simulink model "A3_control_loop_tune"  (Simulink 8.7)
settings: Solver=ode45  StartTime=0.0  StopTime=5.0  MaxStep=1e-3  RelTol=1e-3
values from neighbouring files (symbols this model uses):
  b_1 = 2.39e6    (= 2390000)    [a1_main.m]    (also in a2_main.m; a3_main.m; a4_main.m)
  c_oil = 36.5e6    (= 36500000)    [a1_main.m]    (also in a2_main.m; a3_main.m; a4_main.m)
  c_p = 75e6    (= 75000000)    [a1_main.m]    (also in a2_main.m; a3_main.m; a4_main.m)
  K_M = 1/63000    (= 1.5873015873e-05)    [a1_main.m]    (also in a2_main.m; a3_main.m; a4_main.m)
  m_g = m_k + m_p    (= 268.7)    [a1_main.m]    (also in a2_main.m; a3_main.m; a4_main.m)
libraries: simulink x2
settings Model: Creator=jinyao  LastModifiedBy=jinyao
settings DataIOCC: LimitDataPoints=off  SaveFormat=Dataset
settings DebuggingCC: UnderspecifiedInitializationDetection=Simplified  MergeDetectMultiDrivingBlocksExec=error
settings HardwareCC: ProdBitPerPointer=64  ProdLargestAtomicFloat=Float  ProdIntDivRoundTo=Zero  ProdEndianess=LittleEndian  ProdWordSize=64  ProdHWDeviceType=Intel->x86-64 (Windows64)
settings ModelReferenceCC: PropagateSignalLabelsOutOfModel=on
settings ConfigComp: CovModelRefEnable=off

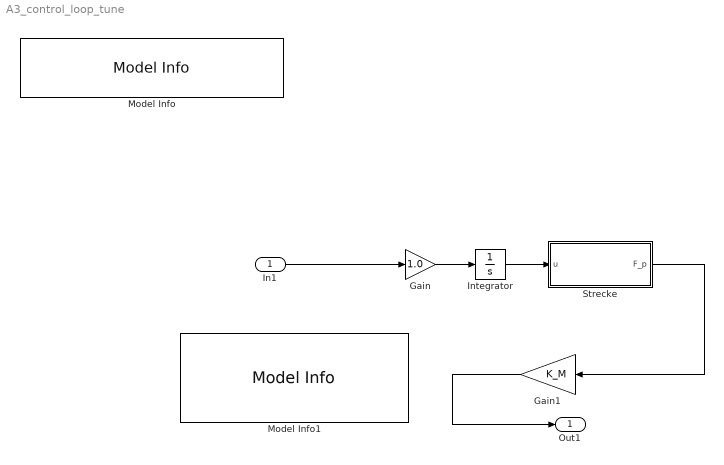
== system A3_control_loop_tune ==
  In1 : Inport
  Gain : Gain  Gain=1.0
  Gain1 : Gain  Gain=K_M
  Integrator : Integrator
  Model Info : simulink/Model-Wide Utilities/Model Info  Frame=on  DisplayStringWithTags=|  HorizontalTextAlignment=Center  LeftAlignmentValue=0.5  SourceBlockDiagram=A3_control_loop_tune  TagMaxNumber=20
      | %<ModelName>
      | 
      | GRUPPE 11
      | 
      | Cao,Bozhi  Gao,Yue  Jia,Xuehua  Zhu,Jinyao
  Model Info1 : simulink/Model-Wide Utilities/Model Info  Frame=on  DisplayStringWithTags=|  HorizontalTextAlignment=Center  LeftAlignmentValue=0.5  SourceBlockDiagram=A3_control_loop_tune  TagMaxNumber=20
      | %<ModelName>
      | 
      | MODSIM GRUPPE 11
      | 
      | Cao,Bozhi  Gao,Yue  Jia,Xuehua  Zhu,Jinyao
      | 
      | 14.06.2018
  Strecke : Subsystem
  Out1 : Outport
  wires:
  Integrator/1 -> Strecke/1(u)
  Gain/1 -> Integrator/1
  In1/1 -> Gain/1
  Strecke/1(F_p) -> Gain1/1
  Gain1/1 -> Out1/1

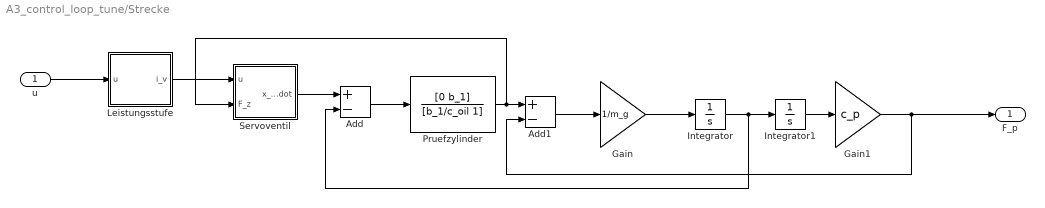
== system A3_control_loop_tune/Strecke ==
  u : Inport
  Add : Sum  Inputs=+-
  Add1 : Sum  Inputs=+-
  Gain : Gain  Gain=1/m_g
  Gain1 : Gain  Gain=c_p
  Integrator : Integrator
  Integrator1 : Integrator
  Leistungsstufe : Subsystem
  Pruefzylinder : TransferFcn  Numerator=[0 b_1]  Denominator=[b_1/c_oil 1]
  Servoventil : Subsystem
  F_p : Outport
  wires:
  Leistungsstufe/1(i_v) -> Servoventil/1(u)
  Servoventil/1(x_oil_dot) -> Add/1
  Add/1 -> Pruefzylinder/1
  Add1/1 -> Gain/1
  Pruefzylinder/1 -> Servoventil/2(F_z), Add1/1
  Gain/1 -> Integrator/1
  Integrator1/1 -> Gain1/1
  Integrator/1 -> Add/2, Integrator1/1
  Gain1/1 -> F_p/1, Add1/2
  u/1 -> Leistungsstufe/1(u)

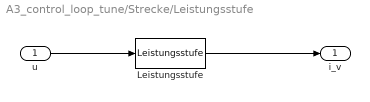
== system A3_control_loop_tune/Strecke/Leistungsstufe ==
  u : Inport
  Leistungsstufe : MATLABFcn  MATLABFcn=Leistungsstufe  OutputDimensions=1  OutputSignalType=real
  i_v : Outport
  wires:
  Leistungsstufe/1 -> i_v/1
  u/1 -> Leistungsstufe/1

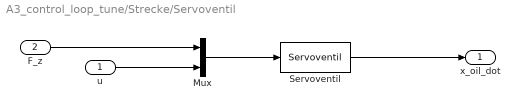
== system A3_control_loop_tune/Strecke/Servoventil ==
  u : Inport
  F_z : Inport  Port=2
  Mux : Mux  Inputs=2
  Servoventil : MATLABFcn  MATLABFcn=Servoventil  OutputDimensions=1  OutputSignalType=real
  x_oil_dot : Outport
  wires:
  Servoventil/1 -> x_oil_dot/1
  u/1 -> Mux/2
  Mux/1 -> Servoventil/1
  F_z/1 -> Mux/1
